simulink library "thermochemical"  (R2017b)
settings: Solver=VariableStepAuto  StartTime=0.0  StopTime=10.0  RelTol=1e-3
values from neighbouring files (symbols this model uses):
  c = conversion_factors()    [blk_clausius_clapeyron.m]    (also in blk_clausius_clapeyron_no_popup.m; blk_cold_room_closed_dry_air.m; blk_reactor_BaCl2_NH3_no_walls.m; blk_reactor_BaCl2_NH3_no_walls_state_space.m)
  cp = metal.cp    [blk_wall_simple.m]    (also in get_metal_properties.m = 390)
  fluid = get_param(blk,'fluid')    [blk_thermodynamic_properties_nonsaturated.m]    (also in blk_thermodynamic_properties_nonsaturated_interpreted.m; blk_thermodynamic_properties_saturated.m; blk_thermodynamic_properties_saturated_interpreted.m; blk_thermodynamic_properties_saturated_mix.m)
  gas = get_material_properties(x.gasName)    [blk_reactor_BaCl2_NH3_cylindrical_no_walls_fun1.m]
  h = get_param(gcb,'ObjectParameters')    [get_param_eval.m]
  rho = metal.rho    [blk_wall_simple.m]    (also in get_metal_properties.m = 8940)
  s = solve(eq,dx,'ReturnConditions',true)    [LMTD_inv.m]    (also in blk_wall_simple.m = get_param_eval(blk,'s'))
  u_gas_at_T_ref = -R * T_ref    [blk_reactor_BaCl2_NH3_no_walls.m]    (also in blk_reactor_BaCl2_NH3_no_walls_state_space.m)
undefined symbols (not defined in the file or in its folder): b_motor, BaCl2, beta, CoolProp, cP_binder, cP_gas, cP_s0, cv, dh_r_0, ENG, heat_exchanger_epsilonNTU_inv_simulink, heat_exchanger_epsilonNTU_simulink, J_motor, K_cin, kappa, Km_motor, La_motor, lookup2D_BreakPoint2, M_binder, N_binder, N_gas_free_volume_init, N_salt, NH3, nh3_v3, nu, P, phase, PID_D_motor, PID_I_motor, PID_P_motor, Ra_motor, Reactor_phase, T, T1, T2, T_init, Tr_init, Tr_ref, U_binder_at_Tr_ref, U_salt_at_X0_Tr_ref, Ur_init, V_void, Valve_regime, Vmax_motor, w_init_motor, X_init
libraries: thermochemical x247, simulink x54, dspsigops x3
(part 2 of 12)

== system thermochemical/Thermodynamic fluid properties ==
  Clausius-Clapeyron : Subsystem  mask(clausius_clapeyron){sel_1=P(T), sel_2=BaCl2/NH3}
      mask prompts: sel_1 "Input/Output"; sel_2 "Pair"
      mask help: Clausius-Clapeyron pressure/temperature relationship for a list of pairs.
      mask init:
      | blk_clausius_clapeyron(gcb)
      mask TypeOptions sel_1: P(T) | T(P)
      mask TypeOptions sel_2: BaCl2/NH3 | NH3(liquid)/NH3(gas)
      mask Display: disp('BaCl2/NH3'); port_label('input',1,'(K)'); port_label('output',1,'(bar)');
  Derivative along saturation curve du/dT (liq.) : Subsystem  mask{fluid=fluid}
      mask prompts: fluid "Thermodynamic properties data (struct variable)"
  Derivative along saturation curve du/dT (vap.) : Subsystem  mask{fluid=fluid}
      mask prompts: fluid "Thermodynamic properties data (struct variable)"
  Derivative along saturation curve dv/dT (liq.) : Subsystem  mask{fluid=fluid}
      mask prompts: fluid "Thermodynamic properties data (struct variable)"
  Derivative along saturation curve dv/dT (vap.) : Subsystem  mask{fluid=fluid}
      mask prompts: fluid "Thermodynamic properties data (struct variable)"
  Derivative in the two-phase region ∂u/∂T|v : Subsystem  mask{fluid=fluid}
      mask prompts: fluid "Thermodynamic properties data (struct variable)"
  Derivative in the two-phase region ∂u/∂v|T : Subsystem  mask{fluid=fluid}
      mask prompts: fluid "Thermodynamic properties data (struct variable)"
  Derivative in the two-phase region ∂χ/∂T|v : Subsystem  mask{fluid=fluid}
      mask prompts: fluid "Thermodynamic properties data (struct variable)"
  Derivative in the two-phase region ∂χ/∂v|T : Subsystem  mask{fluid=fluid}
      mask prompts: fluid "Thermodynamic properties data (struct variable)"
  Enthalpy of ideal gas : Subsystem  mask{T_ref=0, cP_gas=0, h_gas_at_T_ref=0}
      mask prompts: T_ref "Reference temperature [K]"; cP_gas "Ideal gas specific heat at constant pressure Cp [J/K/mol]"; h_gas_at_T_ref "Specific enthalpy at reference temperature h(Tref) [J/mol]"
  Ideal gas equation of state : Subsystem  mask(ideal_gas_equation_of_state){sel=P(T,v), R=8.3145, Pa_to_bar=1e-5, bar_to_Pa=1e5}
      mask prompts: sel "Selection"; R "Universal gas constant [J/K/mol]"; Pa_to_bar "Pa to bar"; bar_to_Pa "bar to Pa"
      mask init:
      | blk_ideal_gas_equation_of_state(gcb)
      mask TypeOptions sel: P(T,v) | P(T,rho) | T(P,v) | T(P,rho) | v(T,P) | rho(T,P)
  Internal energy of ideal gas : Subsystem  mask{T_ref=0, Cv_gas=0, u_gas_at_T_ref=0}
      mask prompts: T_ref "Reference temperature [K]"; Cv_gas "Ideal gas specific heat at constant volume Cv [J/K/mol]"; u_gas_at_T_ref "Specific internal energy at reference temperature u(Tref) [J/mol]"
  Thermodynamic property (non-saturated) : Subsystem  mask(thermodynamic_properties_nonsaturated){sel=v(T,P), fluid=fluid, reciprocVar=+1, lookup2D_BreakPoint1=fluid.no_sat.T_P_indep.var_indep.T, lookup2D_BreakPoint2=fluid.no_sat.T_P_indep.var_indep.P, lookup2D_Data=fluid.no_sat.T_P_indep.var_dep.rho_molar}
      mask prompts: sel "Selection"; fluid "Thermodynamic properties data (struct variable)"
      mask help:
      | The block returns the thermodynamic property of a fluid.
      |
      | The property is chosen from the popup list.
      |
      | The fluid data must be entered as a struct variable.
      |
      | See 'help' for a description of the variables.
      mask init:
      | blk_thermodynamic_properties_nonsaturated(gcb)
      mask Help:
      | The following table describes each symbol:
      | 
      | Symbol	Description			Unit
      | -------------------------------------------------------------------------------
      | T		Temperature						K
      | P		Pressure							bar absolute
      | v		Volume							m3/mol
      | rho		Density							mol/m3
      | u		Internal energy					J/mol
      | h		Enthalpy							J/mol
      | s		Entropy							J/K/mol
      | cp		Specific heat, constant pressure		J/K/mol
      | cv		Specific heat, constant volume		J/K/mol
      | phase	Phase index						See next
      | 
      | The phase  indices are described in the following table:
      | 
      | 0	Subcritical liquid
      | 1	Supercritical (p > pc, T > Tc)
      | 2	Supercritical gas (p < pc, T > Tc)
      | 3	Supercritical liquid (p > pc, T < Tc)
      | 4	At the critical point
      | 5	Subcritical gas
      | 6	Two phase
      | 7	Unknown phase
      | 8	Not imposed
      mask TypeOptions sel: v(T,P) | rho(T,P) | u(T,P) | h(T,P) | s(T,P) | cp(T,P) | cv(T,P) | beta(T,P) | kappa(T,P) | phase(T,P) | T(h,P) | v(h,P) | rho(h,P) | u(h,P) | s(h,P) | cp(h,P) | cv(h,P) | beta(h,P) | kappa(h,P) | phase(h,P) | T(s,P) | v(s,P) | rho(s,P) | u(s,P) | h(s,P) | cp(s,P) | cv(s,P) | beta(s,P) | kappa(s,P) | phase(s,P) | P(T,rho) | u(T,rho) | h(T,rho) | s(T,rho) | cp(T,rho) | cv(T,rho) | beta(T,rho) | kappa(T,rho) | phase(T,rho)
  Thermodynamic property (non-saturated) (it uses CoolProp library) : Subsystem  mask(thermodynamic_properties_nonsaturated_interpreted){sel=v(T,P), fluid=Ammonia, ref=NBP: h=0, s=0 for saturated liquid at 1 atmosphere, reciprocVar=+1}
      mask prompts: sel "Function"; ref "Reference"
      mask help:
      | The block returns the thermodynamic property of a fluid.
      |
      | The property and the fluid are chosen from the popup list.
      |
      | The block uses the CoolProp library, which is called inside a "Interpreted MATLAB Function".
      |
      | See 'help' for a description of the variables and units.
      mask init:
      | blk_thermodynamic_properties_nonsaturated_interpreted(gcb)
      mask Help:
      | The following table describes each symbol:
      | 
      | Symbol	Description			Unit
      | -------------------------------------------------------------------------------
      | T		Temperature						K
      | P		Pressure							bar absolute
      | v		Volume							m3/mol
      | rho		Density							mol/m3
      | u		Internal energy					J/mol
      | h		Enthalpy							J/mol
      | s		Entropy							J/K/mol
      | cp		Specific heat, constant pressure		J/K/mol
      | cv		Specific heat, constant volume		J/K/mol
      | phase	Phase index						See next
      | 
      | The phase  indices are described in the following table:
      | 
      | 0	Subcritical liquid
      | 1	Supercritical (p > pc, T > Tc)
      | 2	Supercritical gas (p < pc, T > Tc)
      | 3	Supercritical liquid (p > pc, T < Tc)
      | 4	At the critical point
      | 5	Subcritical gas
      | 6	Two phase
      | 7	Unknown phase
      | 8	Not imposed
      mask TypeOptions sel: v(T,P) | rho(T,P) | u(T,P) | h(T,P) | s(T,P) | cp(T,P) | cv(T,P) | beta(T,P) | kappa(T,P) | phase(T,P) | T(h,P) | v(h,P) | rho(h,P) | u(h,P) | s(h,P) | cp(h,P) | cv(h,P) | beta(h,P) | kappa(h,P) | phase(h,P) | T(s,P) | v(s,P) | rho(s,P) | u(s,P) | h(s,P) | cp(s,P) | cv(s,P) | beta(s,P) | kappa(s,P) | phase(s,P) | P(T,rho) | u(T,rho) | h(T,rho) | s(T,rho) | cp(T,rho) | cv(T,rho) | beta(T,rho) | kappa(T,rho) | phase(T,rho)
      mask TypeOptions fluid: 1-Butene | Acetone | Air | Air.mix | Amarillo.mix | Ammonia | Argon | Benzene | CarbonDioxide | CarbonMonoxide | CarbonylSulfide | cis-2-Butene | CycloHexane | CycloPropane | Cyclopentane | D4 | D5 | D6 | Deuterium | Dichloroethane | DiethylEther | DimethylCarbonate | DimethylEther | Ekofisk.mix | Ethane | Ethanol | EthylBenzene | Ethylene | EthyleneOxide | Fluorine | GulfCoast.mix | GulfCoastGas(NIST1).mix | HFE143m | HeavyWater | Helium | HighCO2.mix | HighN2.mix | Hydrogen | HydrogenChloride | HydrogenSulfide | IsoButane | IsoButene | Isohexane | Isopentane | Krypton | m-Xylene | MD2M | MD3M | MD4M | MDM | MM | Methane | Methanol | MethylLinoleate | MethylLinolenate | MethylOleate | MethylPalmitate | MethylStearate | n-Butane | n-Decane | n-Dodecane | n-Heptane | n-Hexane | n-Nonane | n-Octane | n-Pentane | n-Propane | n-Undecane | NaturalGasSample.mix | Neon | Neopentane | Nitrogen | NitrousOxide | Novec649 | o-Xylene | OrthoDeuterium | OrthoHydrogen | Oxygen | p-Xylene | ParaDeuterium | ParaHydrogen | Propylene | Propyne | R11 | R113 | R114 | R115 | R116 | R12 | R123 | R1233zd(E) | R1234yf | R1234ze(E) | R1234ze(Z) | R124 | R125 | R13 | R134a | R13I1 | R14 | R141b | R142b | R143a | R152A | R161 | R21 | R218 | R22 | R227EA | R23 | R236EA | R236FA | R245ca | R245fa | R32 | R365MFC | R40 | R401A.mix | R401B.mix | R401C.mix | R402A.mix | R402B.mix | R403A.mix | R403B.mix | R404A | R404A.mix | R405A.mix | R406A.mix | R407A.mix | R407B.mix | R407C | R407C.mix | R407D.mix | R407E.mix | R407F.mix | R408A.mix | R409A.mix | R409B.mix | R41 | R410A | R410A.mix | R410B.mix | R411A.mix | R411B.mix | R412A.mix | R413A.mix | R414A.mix | R414B.mix | R415A.mix | R415B.mix | R416A.mix | R417A.mix | R417B.mix | R417C.mix | R418A.mix | R419A.mix | R419B.mix | R420A.mix | R421A.mix | R421B.mix | R422A.mix | R422B.mix | R422C.mix | R422D.mix | R422E.mix | R423A.mix | R424A.mix | R425A.mix | R426A.mix | R427A.mix | R428A.mix | R429A.mix | R430A.mix | R431A.mix | R432A.mix | R433A.mix | R433B.mix | R433C.mix | R434A.mix | R435A.mix | R436A.mix | R436B.mix | R437A.mix | R438A.mix | R439A.mix | R440A.mix | R441A.mix | R442A.mix | R443A.mix | R444A.mix | R444B.mix | R445A.mix | R446A.mix | R447A.mix | R448A.mix | R449A.mix | R449B.mix | R450A.mix | R451A.mix | R451B.mix | R452A.mix | R453A.mix | R454A.mix | R454B.mix | R500.mix | R501.mix | R502.mix | R503.mix | R504.mix | R507A | R507A.mix | R508A.mix | R508B.mix | R509A.mix | R510A.mix | R511A.mix | R512A.mix | R513A.mix | RC318 | SES36 | SulfurDioxide | SulfurHexafluoride | Toluene | trans-2-Butene | TypicalNaturalGas.mix | Water | Xenon
      mask TypeOptions ref: NBP: h=0, s=0 for saturated liquid at 1 atmosphere | IIR: h = 200 kJ/kg, s=1 kJ/kg/K at 0C saturated liquid | ASHRAE: h = 0, s = 0 @ -40C saturated liquid
  Thermodynamic property (saturated) : Subsystem  mask(thermodynamic_properties_saturated){sel=P(T) (bar), fluid=fluid, lookup1D_BreakPoint1=fluid.sat.T, lookup1D_Data=fluid.sat.Psat}
      mask prompts: sel "Selection"; fluid "Thermodynamic properties data (struct variable)"
      mask help:
      | The block returns the thermodynamic property of a fluid.
      |
      | The property is chosen from the popup list.
      |
      | The fluid data must be entered as a struct variable.
      mask init:
      | blk_thermodynamic_properties_saturated(gcb)
      mask TypeOptions sel: P(T) (bar) | h(T) liq. (J/mol) | h(T) vap. (J/mol) | u(T) liq. (J/mol) | u(T) vap. (J/mol) | s(T) liq. (J/K/mol) | s(T) vap. (J/K/mol) | rho(T) liq. (mol/m3) | rho(T) vap. (mol/m3) | Cp(T) liq. (J/K/mol) | Cp(T) vap. (J/K/mol) | Cv(T) liq. (J/K/mol) | Cv(T) vap. (J/K/mol) | beta(T) liq. (1/K) | beta(T) vap. (1/K) | kappa(T) liq. (1/Pa) | kappa(T) vap. (1/Pa) | T(P) (K) | h(P) liq. (J/mol) | h(P) vap. (J/mol) | u(P) liq. (J/mol) | u(P) vap. (J/mol) | s(P) liq. (J/K/mol) | s(P) vap. (J/K/mol) | rho(P) liq. (mol/m3) | rho(P) vap. (mol/m3) | Cp(P) liq. (J/K/mol) | Cp(P) vap. (J/K/mol) | Cv(P) liq. (J/K/mol) | Cv(P) vap. (J/K/mol) | beta(P) liq. (1/K) | beta(P) vap. (1/K) | kappa(P) liq. (1/Pa) | kappa(P) vap. (1/Pa)
  Thermodynamic property (saturated) (it uses CoolProp library) : Subsystem  mask(thermodynamic_properties_saturated){sel=P(T) (bar), fluid=Ammonia, ref=NBP: h=0, s=0 for saturated liquid at 1 atmosphere, reciprocVar=-1}
      mask prompts: sel "Function"; ref "Reference"
      mask help:
      | The block returns the thermodynamic property of a fluid.
      |
      | The property is chosen from the popup list.
      |
      | The fluid data must be entered as a struct variable.
      mask init:
      | blk_thermodynamic_properties_saturated_interpreted(gcb)
      mask TypeOptions sel: P(T) (bar) | h(T) liq. (J/mol) | h(T) vap. (J/mol) | u(T) liq. (J/mol) | u(T) vap. (J/mol) | s(T) liq. (J/K/mol) | s(T) vap. (J/K/mol) | rho(T) liq. (mol/m3) | rho(T) vap. (mol/m3) | Cp(T) liq. (J/K/mol) | Cp(T) vap. (J/K/mol) | Cv(T) liq. (J/K/mol) | Cv(T) vap. (J/K/mol) | beta(T) liq. (1/K) | beta(T) vap. (1/K) | kappa(T) liq. (1/Pa) | kappa(T) vap. (1/Pa) | T(P) (K) | h(P) liq. (J/mol) | h(P) vap. (J/mol) | u(P) liq. (J/mol) | u(P) vap. (J/mol) | s(P) liq. (J/K/mol) | s(P) vap. (J/K/mol) | rho(P) liq. (mol/m3) | rho(P) vap. (mol/m3) | Cp(P) liq. (J/K/mol) | Cp(P) vap. (J/K/mol) | Cv(P) liq. (J/K/mol) | Cv(P) vap. (J/K/mol) | beta(P) liq. (1/K) | beta(P) vap. (1/K) | kappa(P) liq. (1/Pa) | kappa(P) vap. (1/Pa)
      mask TypeOptions fluid: 1-Butene | Acetone | Air | Air.mix | Amarillo.mix | Ammonia | Argon | Benzene | CarbonDioxide | CarbonMonoxide | CarbonylSulfide | cis-2-Butene | CycloHexane | CycloPropane | Cyclopentane | D4 | D5 | D6 | Deuterium | Dichloroethane | DiethylEther | DimethylCarbonate | DimethylEther | Ekofisk.mix | Ethane | Ethanol | EthylBenzene | Ethylene | EthyleneOxide | Fluorine | GulfCoast.mix | GulfCoastGas(NIST1).mix | HFE143m | HeavyWater | Helium | HighCO2.mix | HighN2.mix | Hydrogen | HydrogenChloride | HydrogenSulfide | IsoButane | IsoButene | Isohexane | Isopentane | Krypton | m-Xylene | MD2M | MD3M | MD4M | MDM | MM | Methane | Methanol | MethylLinoleate | MethylLinolenate | MethylOleate | MethylPalmitate | MethylStearate | n-Butane | n-Decane | n-Dodecane | n-Heptane | n-Hexane | n-Nonane | n-Octane | n-Pentane | n-Propane | n-Undecane | NaturalGasSample.mix | Neon | Neopentane | Nitrogen | NitrousOxide | Novec649 | o-Xylene | OrthoDeuterium | OrthoHydrogen | Oxygen | p-Xylene | ParaDeuterium | ParaHydrogen | Propylene | Propyne | R11 | R113 | R114 | R115 | R116 | R12 | R123 | R1233zd(E) | R1234yf | R1234ze(E) | R1234ze(Z) | R124 | R125 | R13 | R134a | R13I1 | R14 | R141b | R142b | R143a | R152A | R161 | R21 | R218 | R22 | R227EA | R23 | R236EA | R236FA | R245ca | R245fa | R32 | R365MFC | R40 | R401A.mix | R401B.mix | R401C.mix | R402A.mix | R402B.mix | R403A.mix | R403B.mix | R404A | R404A.mix | R405A.mix | R406A.mix | R407A.mix | R407B.mix | R407C | R407C.mix | R407D.mix | R407E.mix | R407F.mix | R408A.mix | R409A.mix | R409B.mix | R41 | R410A | R410A.mix | R410B.mix | R411A.mix | R411B.mix | R412A.mix | R413A.mix | R414A.mix | R414B.mix | R415A.mix | R415B.mix | R416A.mix | R417A.mix | R417B.mix | R417C.mix | R418A.mix | R419A.mix | R419B.mix | R420A.mix | R421A.mix | R421B.mix | R422A.mix | R422B.mix | R422C.mix | R422D.mix | R422E.mix | R423A.mix | R424A.mix | R425A.mix | R426A.mix | R427A.mix | R428A.mix | R429A.mix | R430A.mix | R431A.mix | R432A.mix | R433A.mix | R433B.mix | R433C.mix | R434A.mix | R435A.mix | R436A.mix | R436B.mix | R437A.mix | R438A.mix | R439A.mix | R440A.mix | R441A.mix | R442A.mix | R443A.mix | R444A.mix | R444B.mix | R445A.mix | R446A.mix | R447A.mix | R448A.mix | R449A.mix | R449B.mix | R450A.mix | R451A.mix | R451B.mix | R452A.mix | R453A.mix | R454A.mix | R454B.mix | R500.mix | R501.mix | R502.mix | R503.mix | R504.mix | R507A | R507A.mix | R508A.mix | R508B.mix | R509A.mix | R510A.mix | R511A.mix | R512A.mix | R513A.mix | RC318 | SES36 | SulfurDioxide | SulfurHexafluoride | Toluene | trans-2-Butene | TypicalNaturalGas.mix | Water | Xenon
      mask TypeOptions ref: NBP: h=0, s=0 for saturated liquid at 1 atmosphere | IIR: h = 200 kJ/kg, s=1 kJ/kg/K at 0C saturated liquid | ASHRAE: h = 0, s = 0 @ -40C saturated liquid
  Thermodynamic property (saturated vapor-liquid mix) : Subsystem  mask(thermodynamic_properties_saturated_mix){sel=h(T) (J/mol), fluid=fluid, lookup1D_BreakPoint=0, lookup1D_Data1=fluid.sat.liq.h_molar, lookup1D_Data2=fluid.sat.vap.h_molar}
      mask prompts: sel "Selection"; fluid "Thermodynamic properties data (struct variable)"
      mask help:
      | The block returns the thermodynamic property of a fluid.
      |
      | The property is chosen from the popup list.
      |
      | The fluid data must be entered as a struct variable.
      mask init:
      | blk_thermodynamic_properties_saturated_mix(gcb)
      mask TypeOptions sel: h(T) (J/mol) | u(T) (J/mol) | s(T) (J/K/mol) | rho(T) (mol/m3) | cp(T) (J/K/mol) | cv(T) (J/K/mol)
  Vapor quality & Liquid volumetric fraction : Subsystem  mask{fluid=fluid}
      mask prompts: fluid "Thermodynamic properties data (struct variable)"

== system thermochemical/Thermodynamic processes ==
  Isenthalpic throttling outside saturation dome : Subsystem  mask(isenthalpic_throttling_outside_sat_dome){fluid=fluid}
      mask prompts: fluid "Thermodynamic properties data (struct variable)"
  Mixing chamber (non-saturated) : Subsystem  mask(mixing_chamber_non_saturated){fluid=fluid}
      mask prompts: fluid "Thermodynamic properties data (struct variable)"

== system thermochemical/Utils ==
  "Average computation 1/(T2-T1)*int{x}|t0=T1,tend=T2 (input)" : Subsystem  mask{T1=T1}
      mask prompts: T1 "Integration time window, start time (sec)"
  "Average computation: 1/(T2-T1)*int{x}|t0=T1,tend=T2" : Subsystem  mask{T1=T1, T2=T2}
      mask prompts: T1 "Integration time window, start time (sec)"; T2 "Integration time window, stop time (sec)"

== system thermochemical/Valves ==
  Upstream/downstream detector : Subsystem
  "Valve, gas, IEC 60534-2-1:2012 (exact)" : Subsystem  LoadFcn=|  mask(valve_gas_IEC60534_2_1_exact){Cv_dataPoints=[0 0.01 0.02 0.05 0.09 0.1], apperture_dataPoints=[0 0.2 0.4 0.6 0.8 1], xT=0.5}
      | % For the 'regime' output to work, the model defines an enumerated type:
      | Simulink.defineIntEnumType('Valve_regime',{'Open_NonChocked','Closed','Open_Chocked'},[1 0 -1])
      mask prompts: Cv_dataPoints "Cv vs apperture: Cv data points [0..Cv max]"; apperture_dataPoints "Cv vs apperture: apperture data points [0..1]"; xT "Pressure difference ratio factor of valve without attached fittings at choked flow ('xT' parameter) (use 0.5 if unknown)"
      mask help:
      | Model of a gas flow rate through a valve.
      |
      | The model takes into account the subcritical (non-chocked) and supercritical (chocked) regime of the pressure drop in the valve, switching its behaviour accordingly.
      |
      | The valve apperture is modulated by the signal 'apperture' (apperture = [0..1]).
      |
      | The model expects a table with the values of Cv (flow coeficient) as a function of the valve apperture (0..1).
      | NOTE: the relationship between Cv (imperial units) and Kv (SI units) is: Kv = 0.865*Cv.
      |
      | All the numerical outputs of the model are either positive or zero.
      mask DialogControl Control3 Prompt: Visit SWAGELOK site for more information about valves.
      mask DialogControl Control3 Callback: web('https://www.swagelok.com/en/Resources/CVCalculator','-browser')
  "Valve, gas, IEC 60534-2-1:2012 (modified ideal gas approx.)" : Subsystem  LoadFcn=|  mask(valve_gas_IEC60534_2_1_ideal_gas){Cv_dataPoints=[0 0.01 0.02 0.05 0.09 0.1], apperture_dataPoints=[0 0.2 0.4 0.6 0.8 1], xT=0.5}
      | % For the 'regime' output to work, the model defines an enumerated type:
      | Simulink.defineIntEnumType('Valve_regime',{'Open_NonChocked','Closed','Open_Chocked'},[1 0 -1])
      mask prompts: Cv_dataPoints "Cv vs apperture: Cv data points [0..Cv max]"; apperture_dataPoints "Cv vs apperture: apperture data points [0..1]"; xT "Pressure difference ratio factor of valve without attached fittings at choked flow ('xT' parameter) (use 0.5 if unknown)"
      mask help:
      | Model of a gas flow rate through a valve.
      |
      | The model takes into account the subcritical (non-chocked) and supercritical (chocked) regime of the pressure drop in the valve, switching its behaviour accordingly.
      |
      | The valve apperture is modulated by the signal 'apperture' (apperture = [0..1]).
      |
      | The model expects a table with the values of Cv (flow coeficient) as a function of the valve apperture (0..1).
      | NOTE: the relationship between Cv (imperial units) and Kv (SI units) is: Kv = 0.865*Cv.
      |
      | All the numerical outputs of the model are either positive or zero.
      mask DialogControl Control3 Prompt: Visit SWAGELOK site for more information about valves.
      mask DialogControl Control3 Callback: web('https://www.swagelok.com/en/Resources/CVCalculator','-browser')
  "Valve, gas, Swagelok model" : Subsystem  LoadFcn=|  mask(valve_gas_Swagelok){Cv_dataPoints=[0 0.01 0.02 0.05 0.09 0.1], apperture_dataPoints=[0 0.2 0.4 0.6 0.8 1], rho_gas_60F_1atm_kg_m3=CoolProp.PropsSI('Dmass','T',15.56+273.15,'P',1.0133e5,'Ammonia'), M_gas=CoolProp.Props1SI('M','Ammonia')}
      | % For the 'regime' output to work, the model defines an enumerated type:
      | Simulink.defineIntEnumType('Valve_regime',{'Open_NonChocked','Closed','Open_Chocked'},[1 0 -1])
      mask prompts: Cv_dataPoints "Cv vs apperture: Cv data points [0..Cv max]"; apperture_dataPoints "‘Cv vs apperture: apperture data points [0..1]’"; rho_gas_60F_1atm_kg_m3 "Gas density at 'old' standard condition (60°F, 1atm) (kg/m3)"; M_gas "Gas molar mass (kg/mol)"
      mask help:
      | Model of a gas flow rate through a valve.
      |
      | The model takes into account the subcritical and supercritical regime of the pressure drop in the valve, switching its behaviour accordingly.
      |
      | The valve apperture is modulated by the signal 'apperture' (apperture = [0..1]).
      |
      | The model expects a table with the values of Cv (flow coeficient) as a function of the valve apperture (0..1).
      |
      | NOTE: the relationship between Cv (imperial units) and Kv (SI units) is: Kv = 0.865*Cv.
      |
      | All the numerical outputs of the model are either positive or zero.
      mask DialogControl Control3 Prompt: Visit SWAGELOK site for more information about valves.
      mask DialogControl Control3 Callback: web('https://www.swagelok.com/en/Resources/CVCalculator','-browser')
  "Valve, liquid (chocked condition not implemented)" : Subsystem  LoadFcn=|  mask(valve_liquid){Cv_dataPoints=[0 0.01 0.02 0.05 0.09 0.1], apperture_dataPoints=[0 0.2 0.4 0.6 0.8 1]}
      | % For the 'regime' output to work, the model defines an enumerated type:
      | Simulink.defineIntEnumType('Valve_regime',{'Open_NonChocked','Closed','Open_Chocked'},[1 0 -1])
      mask prompts: Cv_dataPoints "Cv vs apperture: Cv data points [0..Cv max]"; apperture_dataPoints "Cv vs apperture: apperture data points [0..1]"
      mask help:
      | Model of a gas flow rate through a valve.
      |
      | The model assumes turbulent and non-choked flow conditions.
      |
      | The valve apperture is modulated by the signal 'apperture' (apperture = [0..1]).
      |
      | The model expects a table with the values of Cv (flow coeficient) as a function of the valve apperture (0..1).
      |
      | NOTE: the relationship between Cv (imperial units) and Kv (SI units) is: Kv = 0.865*Cv.
      |
      | All the numerical outputs of the model are either positive or zero.
      mask DialogControl Control3 Prompt: Visit SWAGELOK site for more information about valves.
      mask DialogControl Control3 Callback: web('https://www.swagelok.com/en/Resources/CVCalculator','-browser')
  "Valve, liquid, IEC 60534-2-1:2012" : Subsystem  LoadFcn=|  mask(valve_liquid_IEC60534_2_1){Cv_dataPoints=[0 0.01 0.02 0.05 0.09 0.1], apperture_dataPoints=[0 0.2 0.4 0.6 0.8 1], FL=0.74}
      | % For the 'regime' output to work, the model defines an enumerated type:
      | Simulink.defineIntEnumType('Valve_regime',{'Open_NonChocked','Closed','Open_Chocked'},[1 0 -1])
      mask prompts: Cv_dataPoints "Cv vs apperture: Cv data points [0..Cv max]"; apperture_dataPoints "Cv vs apperture: apperture data points [0..1]"; FL "Liquid pressure recovery factor of the valve without attached fittings ('FL' parameter) (≈0.74 for ball valve)"
      mask help:
      | Model of a liquid flow rate through a valve.
      |
      | The model takes into account the subcritical (non-chocked) and supercritical (chocked) regime of the pressure drop in the valve, switching its behaviour accordingly.
      |
      | The valve apperture is modulated by the signal 'apperture' (apperture = [0..1]).
      |
      | The model expects a table with the values of Cv (flow coeficient) as a function of the valve apperture (0..1).
      | NOTE: the relationship between Cv (imperial units) and Kv (SI units) is: Kv = 0.865*Cv.
      |
      | All the numerical outputs of the model are either positive or zero.
      mask DialogControl Control3 Prompt: Visit SWAGELOK site for more information about valves.
      mask DialogControl Control3 Callback: web('https://www.swagelok.com/en/Resources/CVCalculator','-browser')

== system thermochemical/Walls ==
  Fin efficiency : Subsystem  mask(eta_fin){D_mm=100, height_fin_mm=20, thickness_fin_mm=1, lambda=50}
      mask prompts: D_mm "Outer diameter (OD) [mm]"; height_fin_mm "Fin height [mm]"; thickness_fin_mm "Fin thickness [mm]"; lambda "Fin thermal conductivity [W/m/K]"
      mask help:
      | Efficiency equation  for a circular ﬁn of constant cross-section.
      |
      | Ref: Bergman, T. L., and Frank P. Incropera. Fundamentals of heat and mass transfer. Hoboken, NJ: Wiley, 2011. Print. Table 3-5, page 169.
  Radial thermal resistance (no energy accumulation) : Subsystem
  "Wall, simple, h as inputs" : Subsystem  mask(wall_simple){material=Stainless steel, cp=490.8, rho=8023, s=1, e_mm=1, mass=8.023, Twall_init=300}
      mask prompts: cp "Cp [J/K/kg]"; rho "Density [kg/m3]"; s "Surface [m2]"; e_mm "Thickness [mm]"; mass "Mass (for information only) [kg]"; Twall_init "Wall initial condition [K]"
      mask help:
      | Examples of convective heat transfer coeff:
      |   Air, natural convection:	5-10 W/K/m2
      |   Air, forced convection:	100-200 W/K/m2
      mask init:
      | blk_wall_simple(gcb)
      mask TypeOptions material: Aluminum 1100 | Steel | Stainless steel AISI316 | Copper | Custom
      mask Callback material: blk_wall_simple(gcb)
      mask Callback s: blk_wall_simple(gcb)
      mask Callback e_mm: blk_wall_simple(gcb)
  "Wall, tube with/without fins" : Subsystem  mask(wall_finned_tube){L_m=1, OD_mm=10, e_mm=1, material_tube=Aluminum 1100, cp_tube=905.9, rho_tube=2658, height_fin_mm=0, thickness_fin_mm=0, pitch_fin_mm=0, material_fin=Aluminum 1100, cp_fin=905.9, rho_fin=2658, lambda_fin=211.8, Tinit=300, mass_tube=0.075153, mass_fin=0, mass_total=0.075153, s_inner=0.025133, s_outer=0.031416}
      mask prompts: L_m "Length [m]"; OD_mm "Outer diameter (OD) [mm]"; e_mm "Wall thickness [mm]"; material_tube "Material"; cp_tube "Cp [J/K/kg]"; rho_tube "Density [kg/m3]"; height_fin_mm "Fin height [mm]"; thickness_fin_mm "Fin thickness [mm]"; pitch_fin_mm "Fin pitch [mm]"; material_fin "Material"; cp_fin "Cp [J/K/kg]"; rho_fin "Density [kg/m3]"; lambda_fin "Thermal conductivity [J/m/K]"; Tinit "Tube + fins initial temperature [K]"; mass_tube "Bare tube mass [kg]"; mass_fin "Fins mass [kg]"; mass_total "Total mass [kg]"; s_inner "Inner surface [m2]"; s_outer "Outer surface (considering fin effectiveness of 1) [m2]"
      mask help:
      | NOTE: if any of the fin's geometric parameters is zero (e.g. height, width, pitch), a bare tube is considered.
      |
      | Examples of convective heat transfer coeff:
      |   Air, natural convection:	5-10 W/K/m2
      |   Air, forced convection:	100-200 W/K/m2
      mask init:
      | blk_wall_finned_tube(gcb)
      mask TypeOptions material_tube: Aluminum 1100 | Steel | Stainless steel AISI316 | Copper | Custom
      mask Callback material_tube: blk_wall_finned_tube(gcb)
      mask TypeOptions material_fin: Aluminum 1100 | Steel | Stainless steel AISI316 | Copper | Custom
      mask Callback material_fin: blk_wall_finned_tube(gcb)
      mask DialogControl Container5 Prompt: Bare tube
      mask DialogControl Container9 Prompt: Fins
      mask DialogControl Container8 Prompt: Initial conditions
      mask DialogControl Container10 Prompt: Mass and surface (for information only)
  "Wall, tube with/without fins, with internal heat production" : Subsystem  mask(wall_finned_tube){L_m=1, OD_mm=10, e_mm=1, material_tube=Aluminum 1100, cp_tube=905.9, rho_tube=2658, height_fin_mm=0, thickness_fin_mm=0, pitch_fin_mm=0, material_fin=Aluminum 1100, cp_fin=905.9, rho_fin=2658, lambda_fin=211.8, Tinit=300, mass_tube=0.075153, mass_fin=0, mass_total=0.075153, s_inner=0.025133, s_outer=0.031416}
      mask prompts: L_m "Length [m]"; OD_mm "Outer diameter (OD) [mm]"; e_mm "Wall thickness [mm]"; material_tube "Material"; cp_tube "Cp [J/K/kg]"; rho_tube "Density [kg/m3]"; height_fin_mm "Fin height [mm]"; thickness_fin_mm "Fin thickness [mm]"; pitch_fin_mm "Fin pitch [mm]"; material_fin "Material"; cp_fin "Cp [J/K/kg]"; rho_fin "Density [kg/m3]"; lambda_fin "Thermal conductivity [J/m/K]"; Tinit "Tube + fins initial temperature [K]"; mass_tube "Bare tube mass [kg]"; mass_fin "Fins mass [kg]"; mass_total "Total mass [kg]"; s_inner "Inner surface [m2]"; s_outer "Outer surface (considering fin effectiveness of 1) [m2]"
      mask help:
      | NOTE: if any of the fin's geometric parameters is zero (e.g. height, width, pitch), a bare tube is considered.
      |
      | Examples of convective heat transfer coeff:
      |   Air, natural convection:	5-10 W/K/m2
      |   Air, forced convection:	100-200 W/K/m2
      mask init:
      | blk_wall_finned_tube(gcb)
      mask TypeOptions material_tube: Aluminum 1100 | Steel | Stainless steel AISI316 | Copper | Custom
      mask Callback material_tube: blk_wall_finned_tube(gcb)
      mask TypeOptions material_fin: Aluminum 1100 | Steel | Stainless steel AISI316 | Copper | Custom
      mask Callback material_fin: blk_wall_finned_tube(gcb)
      mask DialogControl Container5 Prompt: Bare tube
      mask DialogControl Container9 Prompt: Fins
      mask DialogControl Container8 Prompt: Initial conditions
      mask DialogControl Container10 Prompt: Mass and surface (for information only)

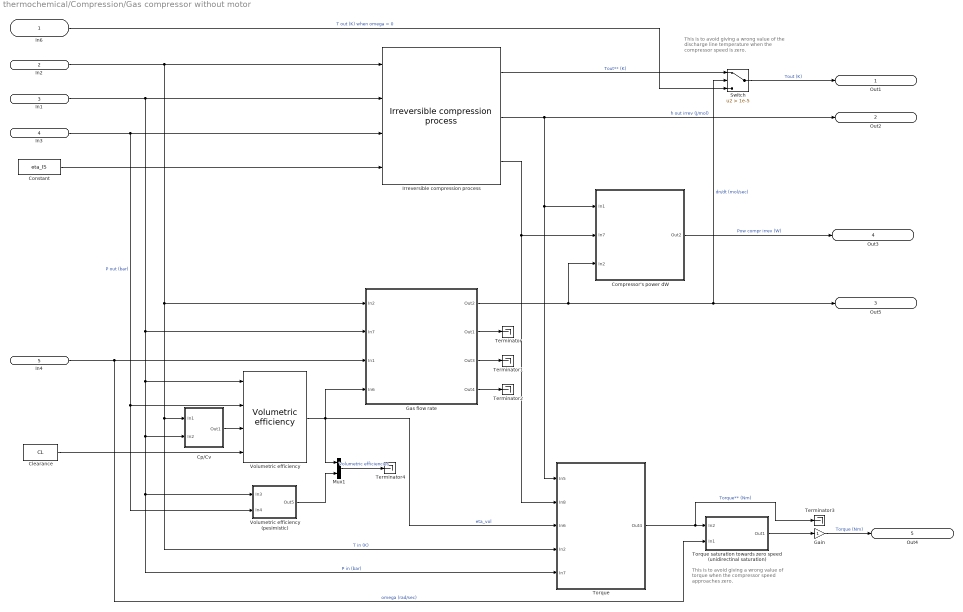
== system thermochemical/Compression/Gas compressor without motor ==
  note: This is to avoid giving a wrong value of
      | the discharge line temperature when
      | the compressor speed is zero.
  note: This is to avoid giving a wrong value
      | of torque when the compressor
      | speed approaches zero.
  In6 : Inport
  In2 : Inport  Port=2
  In1 : Inport  Port=3
  In3 : Inport  Port=4
  In4 : Inport  Port=5
  Clearance : Constant  Value=CL
  Compressor's power dW : Subsystem
  Constant : Constant  Value=eta_IS
  Cp/Cv : Subsystem
  Gain : Gain
  Gas flow rate : Subsystem
  Irreversible compression process : thermochemical/Compression/Irreversible compression process  fluid=fluid
      settings: SourceProductName=@ Thermochemical
  Mux1 : Mux  Inputs=2
  Switch : Switch  Criteria=u2 > Threshold  Threshold=1e-5
  Terminator{,1..4} (5 alike) : Terminator
  "Torque " : Subsystem
  Torque saturation towards zero speed (unidirectinal saturation) : Subsystem  mask(compression_saturation){threshold=0.5, output_min=1e-5}
      mask prompts: threshold "Threshold value (in the units of input)"; output_min "Minimun output value (1e-5 works fine)"
      mask help:
      | The block begins compressing 'input' towards zero when 'control' drops below the programmable threshold.
      |
      | This block is helpful when we need to force a signal go zero when another control variable approaches zero.
      |
      | It replaces a switch block that changes the output to zero when the control signal drops below the threshold. The reason is that the switch block may generate instability.
  Volumetric efficiency : thermochemical/Compression/Volumetric efficiency
      settings: SourceProductName=@ Thermochemical
  Volumetric efficiency (pesimistic) : Subsystem
  Out1 : Outport
  Out2 : Outport  Port=2
  Out5 : Outport  Port=3
  Out3 : Outport  Port=4
  Out4 : Outport  Port=5
  wires:
  Constant/1 -> Irreversible compression process/4
  Switch/1 -> Out1/1  "Tout (K)"
  "Torque "/1(Out4) -> Terminator3/1, Torque saturation towards zero speed (unidirectinal saturation)/1(In2)  "Torque** (Nm)"
  In2/1 -> Irreversible compression process/1, "Torque "/4(In2), Cp/Cv/1(In1), Gas flow rate/1(In2)  "T in (K)"
  Compressor's power dW/1(Out2) -> Out3/1  "Pow compr irrev (W)"
  Volumetric efficiency (pesimistic)/1(Out5) -> Mux1/2
  Volumetric efficiency/1 -> Gas flow rate/4(In6), "Torque "/3(In6), Mux1/1  "eta_vol"
  Gain/1 -> Out4/1  "Torque (Nm)"
  Gas flow rate/1(Out2) -> Compressor's power dW/3(In2), Out5/1, Switch/2  "dn/dt (mol/sec)"
  In3/1 -> Irreversible compression process/3, Volumetric efficiency/2, Volumetric efficiency (pesimistic)/2(In4)  "P out (bar)"
  Irreversible compression process/1 -> Switch/1  "Tout** (K)"
  Mux1/1 -> Terminator4/1  "Volumetric efficiencies"
  In1/1 -> Irreversible compression process/2, Volumetric efficiency/1, Volumetric efficiency (pesimistic)/1(In3), "Torque "/5(In7), Cp/Cv/2(In2), Gas flow rate/2(In7)  "P in (bar)"
  Irreversible compression process/2 -> Compressor's power dW/1(In1), "Torque "/1(In5), Out2/1  "h out irrev (J/mol)"
  Irreversible compression process/3 -> "Torque "/2(In8), Compressor's power dW/2(In7)
  In4/1 -> Torque saturation towards zero speed (unidirectinal saturation)/2(In1), Gas flow rate/3(In1)  "omega (rad/sec)"
  Clearance/1 -> Volumetric efficiency/4
  Cp/Cv/1(Out1) -> Volumetric efficiency/3
  Torque saturation towards zero speed (unidirectinal saturation)/1(Out1) -> Gain/1
  In6/1 -> Switch/3  "T out (K) when omega = 0"
  Gas flow rate/2(Out1) -> Terminator/1
  Gas flow rate/3(Out3) -> Terminator1/1
  Gas flow rate/4(Out4) -> Terminator2/1

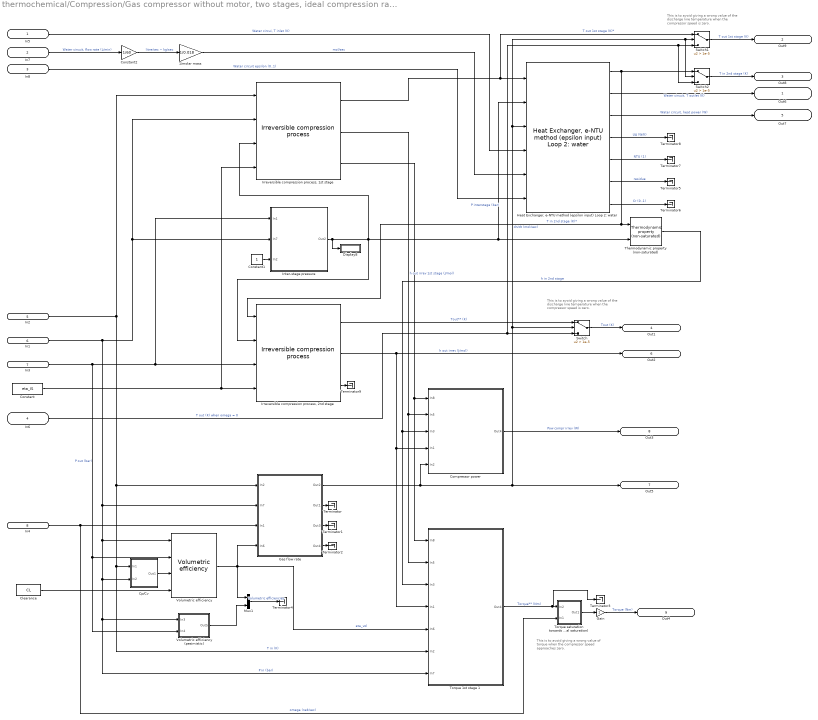
== system thermochemical/Compression/Gas compressor without motor, two stages, ideal compression ratios ==
  note: This is to avoid giving a wrong value of
      | the discharge line temperature when
      | the compressor speed is zero.
  note: This is to avoid giving a wrong value
      | of torque when the compressor
      | speed approaches zero.
  note: This is to avoid giving a wrong value of
      | the discharge line temperature when
      | the compressor speed is zero.
  In5 : Inport
  In7 : Inport  Port=2
  In8 : Inport  Port=3
  In6 : Inport  Port=4
  In2 : Inport  Port=5
  In1 : Inport  Port=6
  In3 : Inport  Port=7
  In4 : Inport  Port=8
  1/molar mass : Gain  Gain=1/0.018
  Clearance : Constant  Value=CL
  Compressor power : Subsystem
  Constant : Constant  Value=eta_IS
  Constant1 : Constant
  Constant2 : Gain  Gain=1/60
  Cp/Cv : Subsystem
  Display8 : Display
  Gain : Gain
  Gas flow rate : Subsystem
  "Heat Exchanger, e-NTU method (epsilon input) Loop 2: water" : thermochemical/Heat exchangers/Heat Exchanger, e-NTU method (epsilon input) Loop 2: water  fluid=fluid  flowType=Counter-flow  cp_water_J_K_mol=75.3260
      settings: SourceProductName=@ Thermochemical
  Inter-stage pressure : Subsystem
  "Irreversible compression process, 1st stage" : thermochemical/Compression/Irreversible compression process  fluid=fluid
      settings: SourceProductName=@ Thermochemical
  "Irreversible compression process, 2nd stage" : thermochemical/Compression/Irreversible compression process  fluid=fluid
      settings: SourceProductName=@ Thermochemical
  Mux1 : Mux  Inputs=2
  Switch : Switch  Criteria=u2 > Threshold  Threshold=1e-5
  Switch1 : Switch  Criteria=u2 > Threshold  Threshold=1e-5
  Switch2 : Switch  Criteria=u2 > Threshold  Threshold=1e-5
  Terminator{,1..9} (10 alike) : Terminator
  Thermodynamic property (non-saturated) : thermochemical/Thermodynamic fluid properties/Thermodynamic  property (non-saturated)  sel=h(T,P)  fluid=fluid  reciprocVar=-1  lookup2D_BreakPoint1=fluid.no_sat.T_P_indep.var_indep.T  lookup2D_BreakPoint2=fluid.no_sat.T_P_indep.var_indep.P  lookup2D_Data=fluid.no_sat.T_P_indep.var_dep.h_molar
      settings: SourceProductName=@ Thermochemical
  Torque 1st stage 1 : Subsystem
  Torque saturation towards zero speed (unidirectinal saturation) : Subsystem  mask(compression_saturation){threshold=0.5, output_min=1e-5}
      mask prompts: threshold "Threshold value (in the units of input)"; output_min "Minimun output value (1e-5 works fine)"
      mask help:
      | The block begins compressing 'input' towards zero when 'control' drops below the programmable threshold.
      |
      | This block is helpful when we need to force a signal go zero when another control variable approaches zero.
      |
      | It replaces a switch block that changes the output to zero when the control signal drops below the threshold. The reason is that the switch block may generate instability.
  Volumetric efficiency : thermochemical/Compression/Volumetric efficiency
      settings: SourceProductName=@ Thermochemical
  Volumetric efficiency (pesimistic) : Subsystem
  Out6 : Outport
  Out9 : Outport  Port=2
  Out8 : Outport  Port=3
  Out1 : Outport  Port=4
  Out7 : Outport  Port=5
  Out2 : Outport  Port=6
  Out5 : Outport  Port=7
  Out3 : Outport  Port=8
  Out4 : Outport  Port=9
  wires:
  Compressor power/1(Out4) -> Out3/1  "Pow compr irrev (W)"
  "Irreversible compression process, 2nd stage"/3 -> Terminator9/1
  In8/1 -> "Heat Exchanger, e-NTU method (epsilon input) Loop 2: water"/6  "Water circuit epsilon (0..1)"
  Constant2/1 -> 1/molar mass/1  "litre/sec ~ kg/sec"
  In7/1 -> Constant2/1  "Water circuit, flow rate (L/min)"
  1/molar mass/1 -> "Heat Exchanger, e-NTU method (epsilon input) Loop 2: water"/5  "mol/sec"
  In5/1 -> "Heat Exchanger, e-NTU method (epsilon input) Loop 2: water"/4  "Water circui, T inlet (K)"
  "Heat Exchanger, e-NTU method (epsilon input) Loop 2: water"/2 -> Out6/1  "Water circuit, T outlet (K)"
  "Heat Exchanger, e-NTU method (epsilon input) Loop 2: water"/3 -> Out7/1  "Water circuit, heat power (W)"
  "Heat Exchanger, e-NTU method (epsilon input) Loop 2: water"/4 -> Terminator8/1  "UA (W/K)"
  "Heat Exchanger, e-NTU method (epsilon input) Loop 2: water"/5 -> Terminator7/1  "NTU (1)"
  "Heat Exchanger, e-NTU method (epsilon input) Loop 2: water"/7 -> Terminator6/1  "Cr (0..1)"
  "Heat Exchanger, e-NTU method (epsilon input) Loop 2: water"/6 -> Terminator5/1  "residue"
  Inter-stage pressure/1(Out2) -> Display8/1, "Irreversible compression process, 2nd stage"/2, Thermodynamic property (non-saturated)/2, "Heat Exchanger, e-NTU method (epsilon input) Loop 2: water"/2, "Irreversible compression process, 1st stage"/3  "P interstage (bar)"
  "Heat Exchanger, e-NTU method (epsilon input) Loop 2: water"/1 -> Switch2/1, Thermodynamic property (non-saturated)/1, "Irreversible compression process, 2nd stage"/1  "T in 2nd stage (K)*"
  Thermodynamic property (non-saturated)/1 -> Torque 1st stage 1/3(In3), Compressor power/3(In3)  "h in 2nd stage"
  Constant1/1 -> Inter-stage pressure/3(In2)
  "Irreversible compression process, 1st stage"/2 -> Torque 1st stage 1/2(In5), Compressor power/2(In5)  "h out irrev 1st stage (J/mol)"
  "Irreversible compression process, 1st stage"/1 -> "Heat Exchanger, e-NTU method (epsilon input) Loop 2: water"/1, Switch1/1  "T out 1st stage (K)*"
  Constant/1 -> "Irreversible compression process, 1st stage"/4, "Irreversible compression process, 2nd stage"/4
  Switch/1 -> Out1/1  "Tout (K)"
  Torque 1st stage 1/1(Out4) -> Terminator3/1, Torque saturation towards zero speed (unidirectinal saturation)/1(In2)  "Torque** (Nm)"
  In2/1 -> Cp/Cv/1(In1), Torque 1st stage 1/6(In2), Gas flow rate/1(In2), "Irreversible compression process, 1st stage"/1  "T in (K)"
  Volumetric efficiency (pesimistic)/1(Out5) -> Mux1/2
  Volumetric efficiency/1 -> Mux1/1, Torque 1st stage 1/5(In6), Gas flow rate/4(In6)  "eta_vol"
  Gain/1 -> Out4/1  "Torque (Nm)"
  Gas flow rate/1(Out2) -> Switch2/2, Switch1/2, "Heat Exchanger, e-NTU method (epsilon input) Loop 2: water"/3, Switch/2, Out5/1, Compressor power/5(In2)  "dn/dt (mol/sec)"
  In3/1 -> Volumetric efficiency/2, Volumetric efficiency (pesimistic)/2(In4), Inter-stage pressure/1(In1), "Irreversible compression process, 2nd stage"/3  "P out (bar)"
  "Irreversible compression process, 2nd stage"/1 -> Switch/1  "Tout** (K)"
  Mux1/1 -> Terminator4/1  "Volumetric efficiencies"
  In1/1 -> Volumetric efficiency/1, Volumetric efficiency (pesimistic)/1(In3), Torque 1st stage 1/7(In7), Cp/Cv/2(In2), Gas flow rate/2(In7), Inter-stage pressure/2(In7), "Irreversible compression process, 1st stage"/2  "P in (bar)"
  "Irreversible compression process, 2nd stage"/2 -> Torque 1st stage 1/4(In1), Compressor power/4(In1), Out2/1  "h out irrev (J/mol)"
  "Irreversible compression process, 1st stage"/3 -> Torque 1st stage 1/1(In8), Compressor power/1(In8)
  In4/1 -> Torque saturation towards zero speed (unidirectinal saturation)/2(In1), Gas flow rate/3(In1)  "omega (rad/sec)"
  Clearance/1 -> Volumetric efficiency/4
  Cp/Cv/1(Out1) -> Volumetric efficiency/3
  Torque saturation towards zero speed (unidirectinal saturation)/1(Out1) -> Gain/1
  In6/1 -> Switch2/3, Switch1/3, Switch/3  "T out (K) when omega = 0"
  Gas flow rate/2(Out1) -> Terminator/1
  Gas flow rate/3(Out3) -> Terminator1/1
  Gas flow rate/4(Out4) -> Terminator2/1
  Switch1/1 -> Out9/1  "T out 1st stage (K)"
  Switch2/1 -> Out8/1  "T in 2nd stage (K)"

== system thermochemical/Compression/Irreversible compression process ==
  note: iseentropic efficiency
  In2 : Inport
  In1 : Inport  Port=2
  In3 : Inport  Port=3
  In4 : Inport  Port=4
  Display6 : Display
  Divide1 : Product  Inputs=*/
  Mux : Mux  Inputs=3
  Sum1 : Sum  Inputs=-+|
  Sum20 : Sum  Inputs=++|
  Terminator : Terminator
  Thermodynamic property (non-saturated) : thermochemical/Thermodynamic fluid properties/Thermodynamic  property (non-saturated)  sel=h(T,P)  fluid=fluid  reciprocVar=-1  lookup2D_BreakPoint1=fluid.no_sat.T_P_indep.var_indep.T  lookup2D_BreakPoint2=fluid.no_sat.T_P_indep.var_indep.P  lookup2D_Data=fluid.no_sat.T_P_indep.var_dep.h_molar
      settings: SourceProductName=@ Thermochemical
  Thermodynamic property (non-saturated)1 : thermochemical/Thermodynamic fluid properties/Thermodynamic  property (non-saturated)  sel=s(T,P)  fluid=fluid  reciprocVar=-1  lookup2D_BreakPoint1=fluid.no_sat.T_P_indep.var_indep.T  lookup2D_BreakPoint2=fluid.no_sat.T_P_indep.var_indep.P  lookup2D_Data=fluid.no_sat.T_P_indep.var_dep.s_molar
      settings: SourceProductName=@ Thermochemical
  Thermodynamic property (non-saturated)2 : thermochemical/Thermodynamic fluid properties/Thermodynamic  property (non-saturated)  sel=h(s,P)  fluid=fluid  reciprocVar=-1  lookup2D_BreakPoint1=fluid.no_sat.s_P_indep.var_indep.s_molar  lookup2D_BreakPoint2=fluid.no_sat.s_P_indep.var_indep.P  lookup2D_Data=fluid.no_sat.s_P_indep.var_dep.h_molar
      settings: SourceProductName=@ Thermochemical
  Thermodynamic property (non-saturated)3 : thermochemical/Thermodynamic fluid properties/Thermodynamic  property (non-saturated)  sel=T(h,P)  fluid=fluid  reciprocVar=-1  lookup2D_BreakPoint1=fluid.no_sat.h_P_indep.var_indep.h_molar  lookup2D_BreakPoint2=fluid.no_sat.h_P_indep.var_indep.P  lookup2D_Data=fluid.no_sat.h_P_indep.var_dep.T
      settings: SourceProductName=@ Thermochemical
  Out1 : Outport
  Out4 : Outport  Port=2
  Out2 : Outport  Port=3
  wires:
  In1/1 -> Thermodynamic property (non-saturated)1/2, Thermodynamic property (non-saturated)/2  "Pin (bar)"
  In3/1 -> Thermodynamic property (non-saturated)3/2, Thermodynamic property (non-saturated)2/2  "Pout (bar)"
  Thermodynamic property (non-saturated)2/1 -> Mux/2, Sum1/2  "h_out rev. (J/mol)"
  Divide1/1 -> Sum20/2
  Sum1/1 -> Divide1/1  "delta h"
  In4/1 -> Divide1/2  "Isentropic efficiency (0..1)"
  Sum20/1 -> Thermodynamic property (non-saturated)3/1, Out4/1, Mux/3  "h out irrev (J/mol)"
  Thermodynamic property (non-saturated)/1 -> Sum1/1, Mux/1, Out2/1, Sum20/1  "h in (J/mol)"
  Thermodynamic property (non-saturated)1/1 -> Thermodynamic property (non-saturated)2/1  "s_out rev.(J/mol/K)"
  Thermodynamic property (non-saturated)3/1 -> Out1/1  "Tout irrev (K)"
  Mux/1 -> Terminator/1, Display6/1  "Enthalpies"
  In2/1 -> Thermodynamic property (non-saturated)1/1, Thermodynamic property (non-saturated)/1  "Tin (K)"

== system thermochemical/Compression/Volumetric efficiency ==
  note: Equation found in:
      | COMPRESSOR HANDBOOK, Paul C. Hanlon (editor),
      | McGRAW-HILL, ISBN 0-07-026005-2
      | Sec. 1.2.5, page 1.11
  In3 : Inport
  In4 : Inport  Port=2
  In1 : Inport  Port=3
  In2 : Inport  Port=4
  Constant : Constant
  Constant1 : Constant
  Divide1 : Product  Inputs=*/
  Divide2 : Product  Inputs=**
  Power : Math  Operator=pow  SaturateOnIntegerOverflow=on
  Recip. : Math  Operator=reciprocal  SaturateOnIntegerOverflow=on
  Saturation : Saturate  UpperLimit=1  LowerLimit=0
  Sum1 : Sum  Inputs=|-+
  Sum2 : Sum  Inputs=|+-
  Out5 : Outport
  wires:
  Sum1/1 -> Saturation/1  "eta vol**"
  Constant/1 -> Sum1/2
  Divide1/1 -> Power/1  "compression_ratio"
  In3/1 -> Divide1/2  "LP (bar)"
  In4/1 -> Divide1/1  "HP (bar)"
  In1/1 -> Recip./1  "Cp/Cv"
  Recip./1 -> Power/2
  Constant1/1 -> Sum2/2
  Power/1 -> Sum2/1
  Sum2/1 -> Divide2/1
  In2/1 -> Divide2/2  "CL (0..1)"
  Divide2/1 -> Sum1/1
  Saturation/1 -> Out5/1  "eta vol"

== system thermochemical/Control volumes/Two-phase saturated fluid control volume (with wall, simple) ==
  In2 : Inport
  In5 : Inport  Port=2
  In6 : Inport  Port=3
  In7 : Inport  Port=4
  In1 : Inport  Port=5
  In3 : Inport  Port=6
  In4 : Inport  Port=7
  In8 : Inport  Port=8
  Gain : Gain  Gain=-1
  Subsystem2 : Subsystem
  Two-phase saturated fluid control volume (without walls) : thermochemical/Control volumes/Two-phase saturated fluid control volume (without walls)  N_init=100  T_init=300  fluid=fluid  V=0.01
      settings: SourceProductName=@ Thermochemical
  "Wall, simple, h as inputs" : thermochemical/Walls/Wall, simple, h as inputs  material=Aluminum 1100  cp=905.9  rho=2658  s=1  e_mm=1  mass=2.658  Twall_init=300
      settings: SourceProductName=@ Thermochemical
  Out6 : Outport
  Out4 : Outport  Port=2
  Out11 : Outport  Port=3
  Out7 : Outport  Port=4
  Out5 : Outport  Port=5
  Out12 : Outport  Port=6
  Out13 : Outport  Port=7
  Out8 : Outport  Port=8
  Out1 : Outport  Port=9
  Out10 : Outport  Port=10
  wires:
  Subsystem2/1(Out1) -> "Wall, simple, h as inputs"/4
  "Wall, simple, h as inputs"/2 -> Gain/1, Out12/1  "q inner → wall (W)"
  "Wall, simple, h as inputs"/1 -> Out11/1  "T wall (K)"
  In3/1 -> "Wall, simple, h as inputs"/2  "h outer (W/m²/K)"
  In4/1 -> Subsystem2/1(In2)  "h inner,liq (W/m²/K)"
  Two-phase saturated fluid control volume (without walls)/7 -> Out1/1  "h liq (sat) (J/mol)"
  Two-phase saturated fluid control volume (without walls)/1 -> "Wall, simple, h as inputs"/3, Out4/1  "T sat (K)"
  Two-phase saturated fluid control volume (without walls)/2 -> Out6/1  "P sat (bar)"
  Two-phase saturated fluid control volume (without walls)/6 -> Out10/1  "h liq+vap (sat) (J/mol)"
  In7/1 -> Two-phase saturated fluid control volume (without walls)/4  "dn/dt vap,out (mol/sec) (must be >= 0 !)"
  Two-phase saturated fluid control volume (without walls)/5 -> Out8/1  "h vap (sat) (J/mol)"
  Two-phase saturated fluid control volume (without walls)/4 -> Out7/1  "vapor quality (0..1)"
  Two-phase saturated fluid control volume (without walls)/3 -> Subsystem2/3(In1), Out5/1  "liquid volumetric fraction (0..1)"
  In5/1 -> Two-phase saturated fluid control volume (without walls)/2  "h in (J/mol)"
  In6/1 -> Two-phase saturated fluid control volume (without walls)/3  "dn/dt in (mol/sec) (must be >= 0 !)"
  In8/1 -> Subsystem2/2(In3)  "h inner,vap (W/m²/K)"
  "Wall, simple, h as inputs"/3 -> Out13/1  "q wall → outer (W)"
  In2/1 -> "Wall, simple, h as inputs"/1  "T outer (K)"
  Gain/1 -> Two-phase saturated fluid control volume (without walls)/1
  In1/1 -> Two-phase saturated fluid control volume (without walls)/5  "dn/dt liq,out (mol/sec) (must be >= 0 !)"
